simulink model "pid_baseline"  (R2024b)
settings: Solver=VariableStepAuto  StartTime=0.0  StopTime=10.0  RelTol=1e-3
values from neighbouring files (symbols this model uses):
  cf = 1.0    (= 1)    [config.m]    (also in controller_config.m = 10; main.m = 10; pid_ga.m = 10)
  de0 = 564.5    [config.m]    (also in controller_config.m; main.m; pid_ga.m)
  de1 = 36.7    [config.m]    (also in controller_config.m; main.m; pid_ga.m)
  de2 = 1    [config.m]    (also in controller_config.m; main.m; pid_ga.m)
  ke = 1.0    (= 1)    [config.m]    (also in controller_config.m = 3000; main.m = 3000; pid_ga.m = 3000)
  ks = 1.0    (= 1)    [config.m]    (also in controller_config.m = 1500; main.m = [0.5, 1.5, 6.0]* 1e3; pid_ga.m = 1500)
  M = 1.0    (= 1)    [config.m]    (also in controller_config.m = 2.9; main.m = 2.9; pid_ga.m = 2.9)
  num0 = 550.5    [config.m]    (also in controller_config.m; main.m; pid_ga.m)
  num1 = -20.15    [config.m]    (also in controller_config.m; main.m; pid_ga.m)
  rg = 1.0    (= 1)    [config.m]    (also in controller_config.m = 0.005; main.m = 0.005; pid_ga.m = 0.005)
libraries: slpidlib x1
settings Model: Creator=hoang  LastModifiedBy=hoang

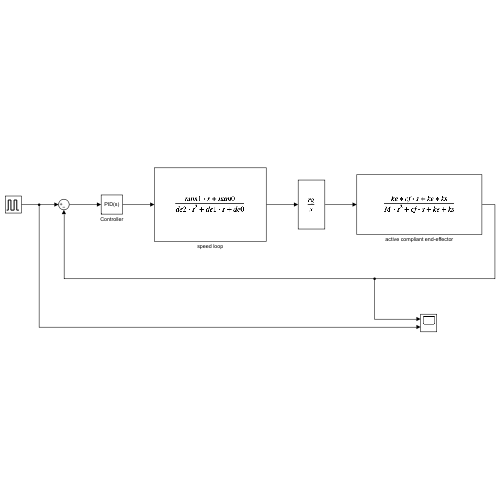
[thumbnail: Simulink's stored preview of the top-level diagram]
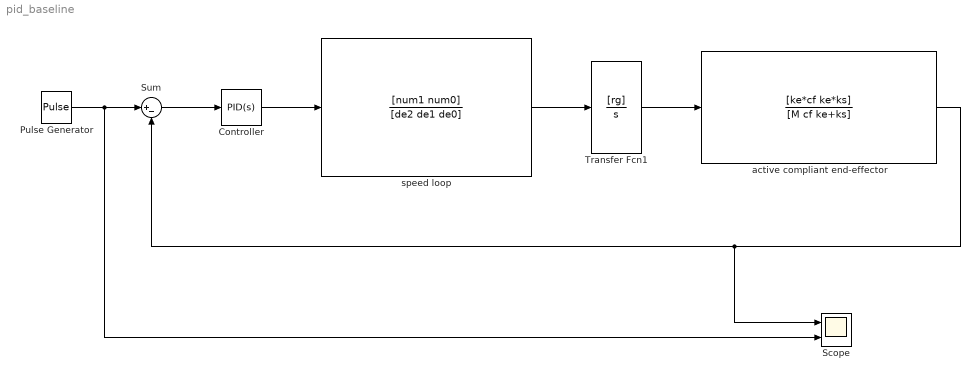
== system pid_baseline ==
  Controller : slpidlib/PID Controller  Controller=PID  Form=Parallel  TimeDomain=Continuous-time  UseExternalTs=off  SampleTime=-1  IntegratorMethod=Forward Euler  FilterMethod=Forward Euler  ControllerParametersSource=internal  P=1.03  I=0.191  UseKiTs=off  D=0.183  UseExternalDerivativeSource=off  N=100  UseFilter=on  TunerSelectOption=Transfer Function Based (PID Tuner App)  InitialConditionSource=internal  InitialConditionForIntegrator=0  InitialConditionForFilter=0  DifferentiatorICPrevScaledInput=0  ExternalReset=none  TrackingMode=off  Kt=1  LimitOutput=off  SatLimitsSource=internal  UpperSaturationLimit=inf  LowerSaturationLimit=-inf  LinearizeAsGain=on  AntiWindupMode=none  Kb=1  LimitIntegrator=off  UpperIntegratorSaturationLimit=inf  LowerIntegratorSaturationLimit=-inf  POutMin=[]  POutMax=[]  IOutMin=[]  IOutMax=[]  DOutMin=[]  DOutMax=[]  NOutMin=[]  NOutMax=[]  SumOutMin=[]  SumOutMax=[]  SaturationOutMin=[]  SaturationOutMax=[]  PParamMin=[]  PParamMax=[]  IParamMin=[]  IParamMax=[]  DParamMin=[]  DParamMax=[]  NParamMin=[]  NParamMax=[]  KbParamMin=[]  KbParamMax=[]  KtParamMin=[]  KtParamMax=[]  KbOutMin=[]  KbOutMax=[]  KtOutMin=[]  KtOutMax=[]  IntegratorOutMin=[]  IntegratorOutMax=[]  FilterOutMin=[]  FilterOutMax=[]  SumI1OutMin=[]  SumI1OutMax=[]  SumI2OutMin=[]  SumI2OutMax=[]  SumI3OutMin=[]  SumI3OutMax=[]  SumI4OutMin=[]  SumI4OutMax=[]  SumDOutMin=[]  SumDOutMax=[]  DifferentiatorOutMin=[]  DifferentiatorOutMax=[]  FilterDiffOutCoefMin=[]  FilterDiffOutCoefMax=[]  ReciprocalOutMin=[]  ReciprocalOutMax=[]  SumDenOutMin=[]  SumDenOutMax=[]  SumNumOutMin=[]  SumNumOutMax=[]  DivideOutMin=[]  DivideOutMax=[]  UdiffTsProdOutMin=[]  UdiffTsProdOutMax=[]  NTsProdOutMin=[]  NTsProdOutMax=[]  UintegralTsProdOutMin=[]  UintegralTsProdOutMax=[]  UngainTsProdOutMin=[]  UngainTsProdOutMax=[]  ClampingZeroOutDataTypeStr=Inherit: Inherit via back propagation  ClampingZeroOutMin=[]  ClampingZeroOutMax=[]  FilterDenConstantOutDataTypeStr=Inherit: Inherit via back propagation  FilterDenConstantOutMin=[]  FilterDenConstantOutMax=[]  PCopyOutDataTypeStr=Inherit: Inherit via back propagation  PCopyOutMin=[]  PCopyOutMax=[]  NCopyOutDataTypeStr=Inherit: Inherit via back propagation  NCopyOutMin=[]  NCopyOutMax=[]  IntegratorContinuousStateAttributes=''  IntegratorStateMustResolveToSignalObject=off  IntegratorRTWStateStorageClass=Auto  FilterContinuousStateAttributes=''  FilterStateMustResolveToSignalObject=off  FilterRTWStateStorageClass=Auto  ParallelPVariant=InternalParameters  IdealPVariant=Disabled  IVariant=InternalParameters  DVariant=InternalParameters  IntegratorVariant=Continuous  SatVariant=Disabled  AWVariant=Passthrough  PCopyVariant=Disabled  TRVariant=Disabled  FdbkBlocksVariant=Forward  IdealPFdbkVariant=Disabled  SatFdbkVariant=Disabled  DerivativeFilterVariant=ContFilter  NVariant=InternalParameters  NCopyVariant=Disabled  FilterICVariant=InternalICsFilter  IntegratorICVariant=InternalICs  ExternalResetVariant=Disabled  TRSumVariant=Passthrough  SumFdbkVariant=Disabled  SumVariant=Sum_PID  TsampFilterVariant=InternalTs  TsampNgainVariant=Passthrough  TsampIntegralVariant=Disabled_SignalSpec  ExternalSaturationOutDataTypeStr=Inherit: Same as second input  DerivativeSourceVariant=ErrorSignal  PreIntVariant=InternalPreInt
  Pulse Generator : DiscretePulseGenerator  PulseType=Time based  Amplitude=10  Period=10  PulseWidth=70  PhaseDelay=01
  Scope : Scope  NumInputPorts=2
  Sum : Sum  Inputs=|+-
  Transfer Fcn1 : TransferFcn  Numerator=[rg]  Denominator=[1 0]
  active compliant end-effector : TransferFcn  Numerator=[ke*cf ke*ks]  Denominator=[M cf ke+ks]
  speed loop : TransferFcn  Numerator=[num1 num0]  Denominator=[de2 de1 de0]
  wires:
  Controller/1 -> speed loop/1
  speed loop/1 -> Transfer Fcn1/1
  Transfer Fcn1/1 -> active compliant end-effector/1
  Sum/1 -> Controller/1
  Pulse Generator/1 -> Scope/2, Sum/1
  active compliant end-effector/1 -> Scope/1, Sum/2
